simulink model "TrafegabilidadeVerticalPassivo"  (R2018a)
settings: Solver=ode3  StartTime=0.0  StopTime=60  FixedStep=0.0001  RelTol=1e-3
values from neighbouring files (symbols this model uses):
  a1 = 1    [Algoritmo_gen.m]    (also in Parametros_dissertacao_Jeff.m = 1.99; custo_gen.m)
  a2 = 100    [Algoritmo_gen.m]    (also in Parametros_dissertacao_Jeff.m = 1.988; custo_gen.m)
  b1 = 0.675    [Parametros_dissertacao_Jeff.m]
  b2 = 0.675    [Parametros_dissertacao_Jeff.m]
  bp1 = 2660    [Parametros_dissertacao_Jeff.m]
  bp2 = 2660    [Parametros_dissertacao_Jeff.m]
  bp3 = 2660    [Parametros_dissertacao_Jeff.m]
  bs1 = 20000    [Parametros_dissertacao_Jeff.m]
  bs2 = 10000    [Parametros_dissertacao_Jeff.m]
  bs3 = 8000    [Parametros_dissertacao_Jeff.m]
  d = 50    [Parametros_dissertacao_Jeff.m]
  fr = 0.01    [Parametros_dissertacao_Jeff.m]
  g = 9.81    [Parametros_dissertacao_Jeff.m]
  h = eig(A_cl2)    [Algoritmo_gen.m]    (also in Parametros_dissertacao_Jeff.m = 0.3; custo_gen.m)
  hcg = 1.359    [Parametros_dissertacao_Jeff.m]
  Ibyy = 66.080    (= 66.08)    [Parametros_dissertacao_Jeff.m]
  Iyy = 284800    [Parametros_dissertacao_Jeff.m]
  kp1 = 770700    [Parametros_dissertacao_Jeff.m]
  kp2 = 770700    [Parametros_dissertacao_Jeff.m]
  kp3 = 770700    [Parametros_dissertacao_Jeff.m]
  ks1 = 59000    [Parametros_dissertacao_Jeff.m]
  ks2 = 3220000    [Parametros_dissertacao_Jeff.m]
  ks3 = 2740000    [Parametros_dissertacao_Jeff.m]
  L = 7    [Parametros_dissertacao_Jeff.m]
  m1 = 490    [Algoritmo_gen.m]    (also in Parametros_dissertacao_Jeff.m; custo_gen.m; n1sistema.m = s(1))
  m2 = 4500    [Algoritmo_gen.m]    (also in Parametros_dissertacao_Jeff.m = 1700; custo_gen.m; n1sistema.m = s(2))
  m3 = 1700    [Parametros_dissertacao_Jeff.m]
  ms = 18470    [Parametros_dissertacao_Jeff.m]
  ms_b = 200    [Parametros_dissertacao_Jeff.m]
  mv = 22560    [Parametros_dissertacao_Jeff.m]
  r_est = 0.542    [Parametros_dissertacao_Jeff.m]
  r_ind = (20*25.4/2+0.5*0.85*395)/1000    (= 0.421875)    [Parametros_dissertacao_Jeff.m]
(part 2 of 2)

== matlab function TrafegabilidadeVerticalPassivo/CHASSIS/TransformcinematicoXZ ==
  data: Fd input; Vd output; Ft input; VCG_Z input; tetap input; Vt1 output; FFcg output; MMcg output
% Sistema de Suspensão - Modelos Passivo e Semiativo
% Autor: Jefferson Gomes de Carvalho Souza
function [Vd,Vt1,FFcg,MMcg]=TransformcinematicoXZ(Fd,Ft,VCG_Z,tetap)
%TC CHASSI
%____________NO PLANO XZ________________
%SAIDAS: vd: Velocidade diantera [m/s]
%________vt: Velocidade traseira [m/s]
%________Fcg: Sumatoria de Forças no CG [N]
%________Mcg: Sumatoria de Momentos em Y mo CG [Nm]
%ENTRDAS:
%________Fd: Força vertical (+Z) eixo dianteiro [N]
%________Ft: Força vertical (+Z) eixo traseiro [N]
%________VCG_Z: Velocidade do centro de gravedade em "Z".
%________Vetor de rotações=[phi,teta,psi]  [rad]
%global a1 a2
a1=2.990; %Comprimento eixo diantero ao CG [m]
a2=1.988; %Comprimento eixo traseiro ao CG [m]
Vc=VCG_Z;
omega=tetap;
%MATRIZ CINEMATICA  PARA TETA < 10°
M_teta_barra=[1 -a1;1 a2];  %[1-a1] matriz teta diantera
                            %[1 a2] matriz teta traseira
                            %Matriz_teta_barra=[M_teta_d;M_teta_t]
V_d_t=[M_teta_barra]*[Vc;omega]; %Matriz de velocidade

Vd=V_d_t(1);    %Velocidade diantera =Primera componente da matriz V_d&t
Vt1=V_d_t(2);    %Velocidade traseira =Segunda Componente da matriz V_d&t

%MATRIZ DINÂMICA
M_teta_barra_trasposta=[M_teta_barra].'; %Matriz trasposta de teta barra
Matriz_Fcg_Mcg=[M_teta_barra_trasposta]*[Fd;Ft];

FFcg=Matriz_Fcg_Mcg(1); %Força no CG = Primeira componente da matriz Matriz_Fcg&Mcg
MMcg=Matriz_Fcg_Mcg(2); %Momento no CG = Primeira componente da matriz Matriz_Fcg&Mcg
                             
end

== matlab function TrafegabilidadeVerticalPassivo/Suspensão batente eixo 3/Z0_Posicao_Solo_3 ==
  data: t input; a2 input; b2 input; d input; L input; h input; Z03 output; vx input
function Z03=fcn(t,a2,b2,d,L,h, vx)

%d:Posição do começo da lombada em [m]
%L:Período da lombada (comprimento entre picos) em [m]
%h: Altura da lombada [m]
%a2: Comprimento desde o cm ao eixo bogie [m]
%b2: Comprimento desde o cm do eixo bogie até o eixo 3[m];
%Ltotal: Comprimento total das lombdas [m]
Ltotal=70; 

Delta_S=vx*t;

%Pneu traseiro
if Delta_S>=(d+a2+b2) && Delta_S<=(d+Ltotal+a2+b2)
    Z03=h*sin(2*pi/L*(vx*t-(d+a2+b2)));
else
    Z03=0;
end

== matlab function TrafegabilidadeVerticalPassivo/Posição XD ==
  data: theta input; XD output; a1 input
function XD = fcn(theta,a1)

XD = a1*cos(theta);
end

== matlab function TrafegabilidadeVerticalPassivo/Posição XT ==
  data: theta input; XT output; a2 input
function XT = fcn(theta,a2)

XT = -a2*cos(theta);
end

== matlab function TrafegabilidadeVerticalPassivo/Posição XT1 ==
  data: theta_bogie input; XT1 output; b1 input
function XT1=fcn(theta_bogie,b1)

XT1 = b1*cos(theta_bogie);
end

== matlab function TrafegabilidadeVerticalPassivo/Posição XT2 ==
  data: theta_bogie input; XT2 output; b2 input
function XT2=fcn(theta_bogie,b2)

XT2 = -b2*cos(theta_bogie);
end

== matlab function TrafegabilidadeVerticalPassivo/MOTOR/T_min [Nm] ==
  data: acel input; T input; Tmot output
function Tmot = fcn(acel, T)
if acel==0
    Tmot=0;
else
    if acel==0.3
    Tmot=33;%35;%100;  %Para 10 khm debe ser T=33 Nm
    else               %Para 20 khm ES MUY rapido!!!!
    Tmot=T;
    end
end
end

== matlab function TrafegabilidadeVerticalPassivo/Rolamento/Fr_ROL_eixo_3 ==
  data: Vv input; W3 input; Fr_ROL_3 output; fr input
function Fr_ROL_3 = fcn(Vv,W3,fr)
%fr:Coeficiente de rolamento
theta=0;% Rampa em grados
%_________________________________________________________%
%____________CONDIÇÃO INICIAL DE ROLAMENTO________________%
if Vv>0   
  %__________FORÇA RESITENTE AO ROLAMENTO___________________%
 Fr_ROL_3 =fr*W3*cos(theta*pi/180);
else
    Fr_ROL_3=0;
end
end

== matlab function TrafegabilidadeVerticalPassivo/Suspensão batente eixo 1/PNEU BATENTE/Batente do pneu ==
  data: deltaZ input; posicao_roda input; posicao_piso input; Fp1 output; kp1 input
% Sistema de Suspensão - Modelos Passivo e Semiativo
% Autor: Jefferson Gomes de Carvalho Souza
function Fp1= fcn(deltaZ, posicao_roda, posicao_piso,kp1)
%% Entradas: deltaZ
%%           
%% Saida: FORÇA DO PNEU [N]
%% ________________________________________________________________________

%kp1=Constante elástica (160000N/m ~ 250000N/m); PNEU(205/50/R15)

Zp=0.1975; %Altura do pneu [m]  (395/85R20)

r_ind=0.4515; %Raio indeformavel[m];  R_ind[m]=r_aro[m]+hp[m]

kp_batente=9e+06; %Faz o pneu rigido.
%%
if deltaZ>=0.95*Zp      %Deflexão maxima.
  
    kp1=kp_batente; %Faz o pneu rigido.

end

if posicao_roda-posicao_piso>r_ind %Perdida de contato
    
    Fp1=0;
else

    Fp1=kp1*deltaZ;%Contato normal
    
end

== matlab function TrafegabilidadeVerticalPassivo/Suspensão batente eixo 1/SUSPENSÃO BATENTE/Batente da suspensão ==
  data: ks1 input; DeltaZ input; FK1 output
% Sistema de Suspensão - Modelos Passivo e Semiativo
% Autor: Jefferson Gomes de Carvalho Souza
function FK1 = fcn(ks1, DeltaZ)
%% Entradas: DeltaZ(Z1-Zd) [m] e Zd [m] parte diantera.
%% MOLA
%MOLA SUSPENSÃO   [ks] (10000Nm ~ 20000Nm)
%km_rebound=1e+06;  
%REBOUND:Constante elástica de mola no caso a roda esteja sem contato.
km_bump=1.5e+06; %BUMP:Constante elástica máxima da mola. 
delta_max=0.7;
if DeltaZ<=delta_max
    FK1=ks1*DeltaZ;
else
    FK1=km_bump*DeltaZ;
end

== matlab function TrafegabilidadeVerticalPassivo/Suspensão batente eixo 1/Z0_Posicao_Solo_1 ==
  data: t input; a1 input; d input; L input; h input; Z01 output; vx input
function Z01= fcn(t,a1,d,L,h,vx)

%d: Posição do começo da lombada em [m]
%L: Período da lombada (comprimento entre picos) em [m]
%h: Altura da lombada [m]
%a1:Comprimento desde o cm ao eixo dianteiro [m]
%Ltotal: Comprimento da lombada [m]
Ltotal=70; 

Delta_S=vx*t;

%Pneu dianteiro
if Delta_S>=(d-a1) && Delta_S<=(d+Ltotal-a1)
    Z01=h*sin(2*pi/L*(vx*t-(d-a1)));
else
    Z01=0;
 end

== matlab function TrafegabilidadeVerticalPassivo/Suspensão batente eixo 2/PNEU BATENTE/Batente do pneu ==
  data: deltaZ input; posicao_roda input; posicao_piso input; Fp2 output; kp2 input
function Fp2= fcn(deltaZ, posicao_roda, posicao_piso,kp2)
%% Entradas: deltaZ
%%           
%% Saida: FORÇA DO PNEU [N]
%% ________________________________________________________________________

%kp2=Constante elástica (160000N/m ~ 250000N/m); PNEU(205/50/R15)

Zp=0.1975; %Altura do pneu [m]  (395/85R20)

r_ind=0.4515; %Raio indeformavel[m];  R_ind[m]=r_aro[m]+hp[m]

kp_batente=9e+06; %Faz o pneu rigido.
%%
if deltaZ>=0.95*Zp      %Deflexão maxima.
  
    kp2=kp_batente; %Faz o pneu rigido.

end

if posicao_roda-posicao_piso>r_ind %Perdida de contato
    
    Fp2=0;
    
else

    Fp2=kp2*deltaZ;%Contato normal
    
end

== matlab function TrafegabilidadeVerticalPassivo/Suspensão batente eixo 2/SUSPENSÃO BATENTE/Batente da suspensão ==
  data: ks2 input; DeltaZ input; FK2 output
function FK2 = fcn(ks2, DeltaZ)
%% Entradas: DeltaZ(Z2-ZT1) [m] e ZT1 [m] parte traseira.
%% MOLA
%MOLA SUSPENSÃO   [ks] (10000Nm ~ 20000Nm)
%km_rebound=1e+06;   
%REBOUND:Constante elástica de mola no caso a roda esteja sem contato.
km_bump=1.5e+06; %BUMP:Constante elástica máxima da mola. 
delta_max=0.7;
if DeltaZ<=delta_max
    FK2=ks2*DeltaZ;
else
    FK2=km_bump*DeltaZ;
end

== matlab function TrafegabilidadeVerticalPassivo/Suspensão batente eixo 2/Z0_Posicao_Solo_2 ==
  data: t input; a2 input; b1 input; d input; L input; h input; Z02 output; vx input
function Z02= fcn(t,a2,b1,d,L,h,vx)

%d:Posição do começo da lombada em [m]
%L:Período da lombada (comprimento entre picos) em [m]
%h:Altura da lombada [m]
%a2: Comprimento desde o cm ao eixo centro do bogie [m]
%b1: Comprimento desde o cm do bogie ao eixo 2.[m]
%Ltotla: compriemento das lombadas [m]
Ltotal=70; 

Delta_S=vx*t;

%Pneu traseiro
if Delta_S>=(d+a2-b1) && Delta_S<=(d+Ltotal+a2-b1) 
    Z02=h*sin(2*pi/L*(vx*t-(d+a2-b1)));
else
    Z02=0;
end

== matlab function TrafegabilidadeVerticalPassivo/Matriz de transformação do perfil do chassis ==
  data: Xcg input; PF1 output; Zcg input; theta input; PF2 output; PF3 output; PF4 output; PF5 output; PF6 output; PF7 output; PF8 output
function [PF1,PF2,PF3,PF4,PF5,PF6,PF7,PF8] = fcn(Xcg,Zcg,theta)
 
a1=3.42; %Comprimento eixo diantero ao CG [m]
a2=1.35; %Comprimento eixo tras eiro ao CG [m]
 
P1=[-a2-1.5;0;-0.2-0.3];
P2=[a1+1.3;0;-0.2-0.3];
P3=[a1+1.5;0;0-0.3];
P4=[a1+1.5;0;0.5617-0.3];
P5=[a1+1.4;0;1.40-0.3];
P6=[3;0;1.40-0.3];
P7=[2.9;0;0.2-0.3];
P8=[-a2-1.5;0;0.2-0.3];

%Matriz de transformação  
T=[cos(theta),0,-sin(theta);0,1,0;sin(theta),0,cos(theta)];
PF1=[Xcg;0;Zcg]+T*P1;
PF2=[Xcg;0;Zcg]+T*P2;
PF3=[Xcg;0;Zcg]+T*P3;
PF4=[Xcg;0;Zcg]+T*P4;
PF5=[Xcg;0;Zcg]+T*P5;
PF6=[Xcg;0;Zcg]+T*P6;
PF7=[Xcg;0;Zcg]+T*P7;
PF8=[Xcg;0;Zcg]+T*P8;

== matlab function TrafegabilidadeVerticalPassivo/BOGIE/TransformcinematicoXZ ==
  data: Fd input; Vd output; Ft input; VCG_Z input; tetap input; Vt1 output; FFcg output; MMcg output
% Sistema de Suspensão - Modelos Passivo e Semiativo
% Autor: Jefferson Gomes de Carvalho Souza
function [Vd,Vt1,FFcg,MMcg]=TransformcinematicoXZ(Fd,Ft,VCG_Z,tetap)
%TC BOGIE
%____________NO PLANO XZ________________
%SAIDAS: vd: Velocidade diantera [m/s]
%________vt: Velocidade traseira [m/s]
%________Fcg: Sumatoria de Forças no CG [N]
%________Mcg: Sumatoria de Momentos em Y mo CG [Nm]
%ENTRDAS:
%________Fd: Força vertical (+Z) eixo dianteiro [N]
%________Ft: Força vertical (+Z) eixo traseiro [N]
%________VCG_Z: Velocidade do centro de gravedade em "Z".
%________Vetor de rotações=[phi,teta,psi]  [rad]

b1=0.675;
b2=0.675;
Vc=VCG_Z;
omega=tetap;
%MATRIZ CINEMATICA  PARA TETA < 10°
M_teta_barra=[1 -b1;1 b2];  %[1-a1] matriz teta diantera
                            %[1 a2] matriz teta traseira
                            %Matriz_teta_barra=[M_teta_d;M_teta_t]
V_d_t=[M_teta_barra]*[Vc;omega]; %Matriz de velocidade

Vd=V_d_t(1);    %Velocidade diantera =Primera componente da matriz V_d&t
Vt1=V_d_t(2);    %Velocidade traseira =Segunda Componente da matriz V_d&t

%MATRIZ DINÂMICA
M_teta_barra_trasposta=[M_teta_barra].'; %Matriz trasposta de teta barra
Matriz_Fcg_Mcg=[M_teta_barra_trasposta]*[Fd;Ft];

FFcg=Matriz_Fcg_Mcg(1); %Força no CG = Primeira componente da matriz Matriz_Fcg&Mcg
MMcg=Matriz_Fcg_Mcg(2); %Momento no CG = Primeira componente da matriz Matriz_Fcg&Mcg
                             
end

== matlab function TrafegabilidadeVerticalPassivo/Motorista/Limitador de marcha ==
  data: m input; marcha output; v input
function marcha = fcn(m,v)
if v==10%15
    marcha=4;%7
else
    marcha=m;
end
